simulink model "Three_Phase_Full_Wave_Bridge_Rectifier"  (R2018a)
settings: Solver=VariableStepAuto  StartTime=0.0  StopTime=0.1  RelTol=1e-3
libraries: powerlib x31, powerlib_meascontrol x5
settings Model: Creator=ozie  LastModifiedBy=ozie

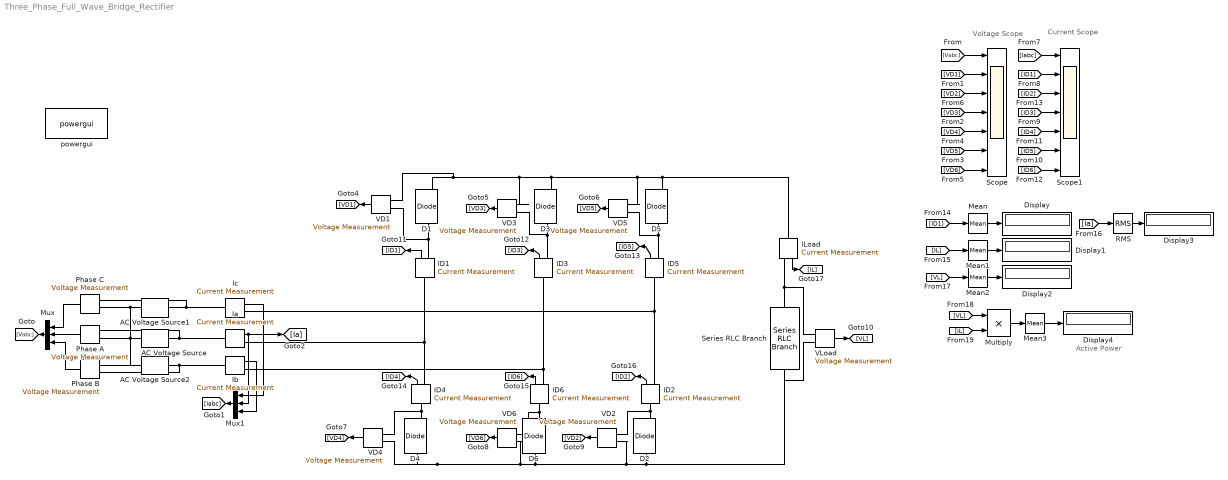
== system Three_Phase_Full_Wave_Bridge_Rectifier ==
  note: Active Power
  note: Current Scope
  note: Voltage Scope
  AC Voltage Source : powerlib/Electrical Sources/AC Voltage Source  Amplitude=220*sqrt(2)  Phase=0  Frequency=50  SampleTime=0  Measurements=None  BusType=swing  Pref=10e3  Qref=0  Qmin=-inf  Qmax=+inf
  AC Voltage Source1 : powerlib/Electrical Sources/AC Voltage Source  Amplitude=220*sqrt(2)  Phase=-120  Frequency=50  SampleTime=0  Measurements=None  BusType=swing  Pref=10e3  Qref=0  Qmin=-inf  Qmax=+inf
  AC Voltage Source2 : powerlib/Electrical Sources/AC Voltage Source  Amplitude=220*sqrt(2)  Phase=120  Frequency=50  SampleTime=0  Measurements=None  BusType=swing  Pref=10e3  Qref=0  Qmin=-inf  Qmax=+inf
  D{1..6} (6 alike) : powerlib/Power Electronics/Diode  Ron=0.001  Lon=0  Vf=0.8  IC=0  UseSnubber=0  Rs=500  Cs=250e-9  Measurements=on
  Display{,1..4} (5 alike) : Display
      Display4 settings: Format=bank
  ID{1..6} (6 alike) : powerlib/Measurements/Current Measurement  PhasorSimulation=off  OutputType=Complex  PSBequivalent=0
  ILoad : powerlib/Measurements/Current Measurement  PhasorSimulation=off  OutputType=Complex  PSBequivalent=0
  Ia : powerlib/Measurements/Current Measurement  PhasorSimulation=off  OutputType=Complex  PSBequivalent=0
  Ib : powerlib/Measurements/Current Measurement  PhasorSimulation=off  OutputType=Complex  PSBequivalent=0
  Ic : powerlib/Measurements/Current Measurement  PhasorSimulation=off  OutputType=Complex  PSBequivalent=0
  Mean{,1..3} (4 alike) : powerlib_meascontrol/Measurements/Mean  Freq=50  Vinit=0  Ts=0
  Multiply : Product
  Mux : Mux  Inputs=3
      settings: DisplayOption=signals
  Mux1 : Mux  Inputs=3
      settings: DisplayOption=signals
  "Phase A " : powerlib/Measurements/Voltage Measurement  PhasorSimulation=off  OutputType=Complex  PSBequivalent=0
  "Phase B " : powerlib/Measurements/Voltage Measurement  PhasorSimulation=off  OutputType=Complex  PSBequivalent=0
  Phase C : powerlib/Measurements/Voltage Measurement  PhasorSimulation=off  OutputType=Complex  PSBequivalent=0
  RMS : powerlib_meascontrol/Measurements/RMS  TrueRMS=on  Freq=50  RMSInit=120  Ts=0
  Scope : Scope  NumInputPorts=7
  Scope1 : Scope  NumInputPorts=7
  Series RLC Branch : powerlib/Elements/Series RLC Branch  LConnTagsString=__new0  RConnTagsString=__new0  BranchType=RL  Resistance=10  Inductance=20e-3  SetiL0=off  InitialCurrent=0  Capacitance=1e-6  Setx0=off  InitialVoltage=0  Measurements=None
  VD{1..6} (6 alike) : powerlib/Measurements/Voltage Measurement  PhasorSimulation=off  OutputType=Complex  PSBequivalent=0
  VLoad : powerlib/Measurements/Voltage Measurement  PhasorSimulation=off  OutputType=Complex  PSBequivalent=0
  powergui : powerlib/powergui  Priority=1  SimulationMode=Continuous  SampleTime=50e-6  frequency=60  Iterations=50  frequencyindice=50  Pbase=100e6  ErrMax=1e-4  UnitsV=kV  UnitsW=MW  buscounter=0  FunctionMessages=off  echomessages=off  EnableUseOfTLC=off  CurrentSourceSwitches=off  DisableSnubberDevices=off  DisableRonSwitches=off  DisableVfSwitches=off  DisplayEquations=off  SolverType=Tustin/Backward Euler (TBE)  Interpol=off  ExternalGateDelay=off  methode=off  Ts=100  x0status=blocks  SPID=on  SwTol=0  HookPort=off  RestoreLinks=warning  ResistiveCurrentMeasurement=off  Frange=[0:2:500]  Ylog=off  Xlog=on  ShowGrid=off  save=off  variable=ZData  structure=0  ZoomFFT=off  StartTime=0.0  cycles=1  DisplayStyle=1  fundamental=60  FreqAxis=off  MaxFrequency=1000  frequencyindicesteady=1  RmsSteady=1  display=off
  wires:
  Phase C/1 -> Mux/1
  "Phase A "/1 -> Mux/2
  "Phase B "/1 -> Mux/3
  Mux/1 -> [Vabc]
  Ia/1 -> [Ia], Mux1/2
  Ib/1 -> Mux1/3
  VD1/1 -> [VD1]
  VD3/1 -> [VD3]
  VD5/1 -> [VD5]
  VD4/1 -> [VD4]
  VD6/1 -> [VD6]
  VD2/1 -> [VD2]
  VLoad/1 -> [VL]
  ID1/1 -> [ID1]
  ID3/1 -> [ID3]
  ID5/1 -> [ID5]
  ID4/1 -> [ID4]
  ID6/1 -> [ID6]
  ID2/1 -> [ID2]
  ILoad/1 -> [IL]
  [Vabc] -> Scope/1
  [VD2] -> Scope/3
  [VD6] -> Scope/7
  Ic/1 -> Mux1/1
  Mux1/1 -> [Iabc]
  [Iabc] -> Scope1/1
  [VD3] -> Scope/4
  [VD4] -> Scope/5
  [VD5] -> Scope/6
  [VD1] -> Scope/2
  [ID1] -> Scope1/2
  [ID2] -> Scope1/3
  [ID3] -> Scope1/4
  [ID4] -> Scope1/5
  [ID5] -> Scope1/6
  [ID6] -> Scope1/7
  [ID1] -> Mean/1
  [IL] -> Mean1/1
  [Ia] -> RMS/1
  [VL] -> Mean2/1
  Mean/1 -> Display/1
  Mean1/1 -> Display1/1
  Mean2/1 -> Display2/1
  RMS/1 -> Display3/1
  [VL] -> Multiply/1
  [IL] -> Multiply/2
  Multiply/1 -> Mean3/1
  Mean3/1 -> Display4/1
  connections:
  AC Voltage Source1/LConn1 -- "Phase B "/LConn2 -- AC Voltage Source2/LConn1 -- AC Voltage Source/LConn1 -- "Phase A "/LConn2 -- Phase C/LConn2
  Ia/RConn1 -- ID1/LConn1 -- ID4/RConn1
  AC Voltage Source2/RConn1 -- "Phase B "/LConn1 -- Ib/LConn1
  AC Voltage Source1/RConn1 -- Phase C/LConn1 -- Ic/LConn1
  D2/LConn1 -- VLoad/LConn2 -- Series RLC Branch/RConn1 -- VD2/LConn1 -- D6/LConn1 -- VD6/LConn1 -- D4/LConn1 -- VD4/LConn1
  D1/RConn1 -- VD1/LConn2 -- VD3/LConn2 -- VD5/LConn2 -- ILoad/LConn1 -- D5/RConn1 -- D3/RConn1
  D5/LConn1 -- VD5/LConn1 -- ID5/RConn1
  AC Voltage Source/RConn1 -- "Phase A "/LConn1 -- Ia/LConn1
  ID3/LConn1 -- ID6/RConn1 -- Ib/RConn1
  D1/LConn1 -- VD1/LConn1 -- ID1/RConn1
  D3/LConn1 -- VD3/LConn1 -- ID3/RConn1
  Ic/RConn1 -- ID5/LConn1 -- ID2/RConn1
  ILoad/RConn1 -- VLoad/LConn1 -- Series RLC Branch/LConn1
  ID4/LConn1 -- VD4/LConn2 -- D4/RConn1
  ID6/LConn1 -- VD6/LConn2 -- D6/RConn1
  ID2/LConn1 -- VD2/LConn2 -- D2/RConn1
